simulink model "Controlador_por_retro_de_error"  (R2022b)
settings: Solver=VariableStepAuto  StartTime=0.0  StopTime=10.0  RelTol=1e-3
InitFcn:
  | Ke = -3;
  | k=0.5;
  | b=1;
  | M = 1;
  | 
  | A = [0 1; -k/M -b/M; ];
  | B = [0;1/M];
  | C = [1,0;0,1];
settings Model: Creator=garci  LastModifiedBy=garci

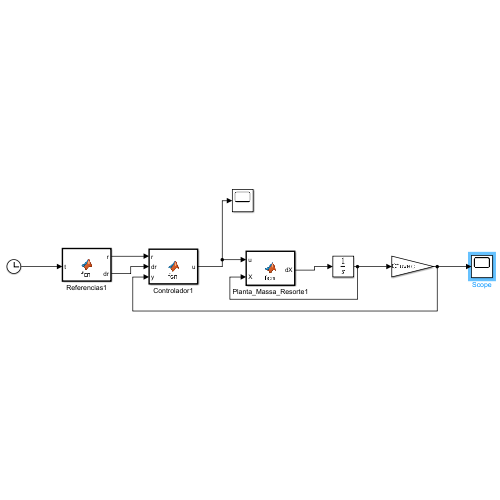
[thumbnail: Simulink's stored preview of the top-level diagram]
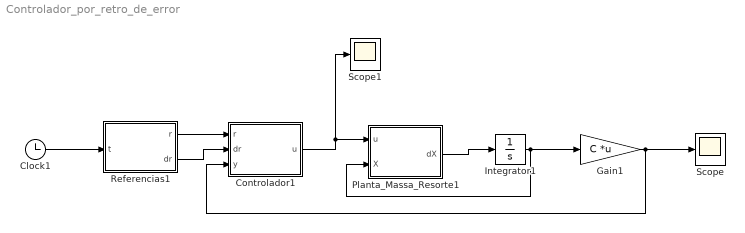
== system Controlador_por_retro_de_error ==
  Clock1 : Clock
  Controlador1 : MATLAB Function  TreatAsAtomicUnit=on
  Gain1 : Gain  Gain=C  Multiplication=Matrix(K*u) (u vector)
  Integrator1 : Integrator
  Planta_Massa_Resorte1 : MATLAB Function  TreatAsAtomicUnit=on
  Referencias1 : MATLAB Function  TreatAsAtomicUnit=on
  Scope : Scope
  Scope1 : Scope
  wires:
  Clock1/1 -> Referencias1/1(t)
  Referencias1/1(r) -> Controlador1/1(r)
  Referencias1/2(dr) -> Controlador1/2(dr)
  Controlador1/1(u) -> Scope1/1, Planta_Massa_Resorte1/1(u)
  Planta_Massa_Resorte1/1(dX) -> Integrator1/1
  Integrator1/1 -> Planta_Massa_Resorte1/2(X), Gain1/1
  Gain1/1 -> Controlador1/3(y), Scope/1

== matlab function Controlador_por_retro_de_error/Controlador1 ==
  data: r input; u output; dr input; y input; Ke parameter; C parameter; A parameter; B parameter
function u = fcn(r, dr, y, Ke, C, A, B)

X = y; %recuperar estados de las salidas
C2 = C(2,:); %salida a controlar
y2 = C2*X; %definiendo salida a controlar 
e = r- y2; %Variable de error
u = (C2*B)^-1 * (dr- C2*A*X -Ke*e); %señal de control

== matlab function Controlador_por_retro_de_error/Planta_Massa_Resorte1 ==
  data: u input; dX output; X input; A parameter; B parameter
function dX = fcn(u, X, A, B)

dX = A*X + B*u;

== matlab function Controlador_por_retro_de_error/Referencias1 ==
  data: t input; r output; dr output
function [r, dr] = fcn(t)

r = 2 + sin(t);
dr = cos(t);
